simulink model "TestConnectors"  (Simulink 7.8)
settings: Solver=ode45  StartTime=0.0  StopTime=10.0  RelTol=1e-3
settings Model: Creator=PtheG  LastModifiedBy=Pedram Nazari

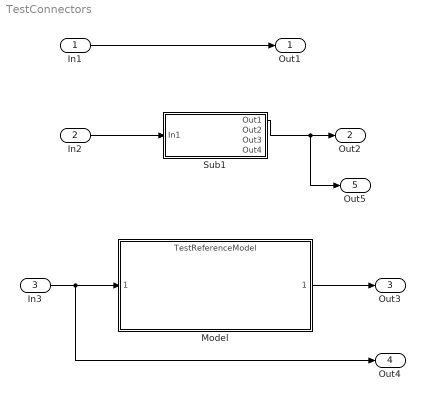
== system TestConnectors ==
  In1 : Inport
  In2 : Inport  Port=2
  In3 : Inport  Port=3
  Model : ModelReference  ModelNameDialog=TestReferenceModel  SimulationMode=Normal  ModelReferenceVersion=1.1  CopyOfModelName=TestReferenceModel  DefaultDataLogging=on
  Sub1 : Subsystem
  Out1 : Outport
  Out2 : Outport  Port=2
  Out3 : Outport  Port=3
  Out4 : Outport  Port=4
  Out5 : Outport  Port=5
  wires:
  In2/1 -> Sub1/1(In1)
  In3/1 -> Model/1, Out4/1
  Model/1 -> Out3/1
  Sub1/1(Out1) -> Out2/1, Out5/1
  In1/1 -> Out1/1

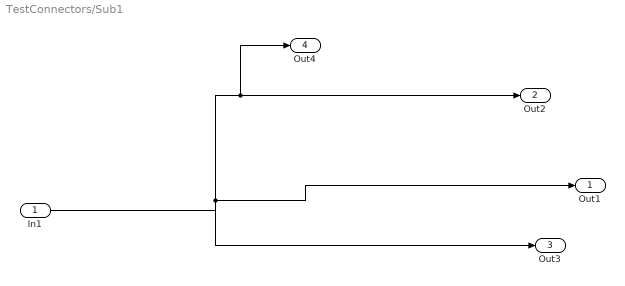
== system TestConnectors/Sub1 ==
  In1 : Inport
  Out1 : Outport
  Out2 : Outport  Port=2
  Out3 : Outport  Port=3
  Out4 : Outport  Port=4
  wires:
  In1/1 -> Out1/1, Out3/1, Out2/1, Out4/1
